simulink model "Channel_estimation_working1"  (R2016b)
settings: Solver=VariableStepAuto  StartTime=0.0  StopTime=10.0  RelTol=1e-3
undefined symbols (not defined in the file or in its folder): physconst
libraries: phasedtxrxlib x7, phasedenvlib x4, dspinverses x2
settings Model: Creator=CHAITRA  LastModifiedBy=ishu

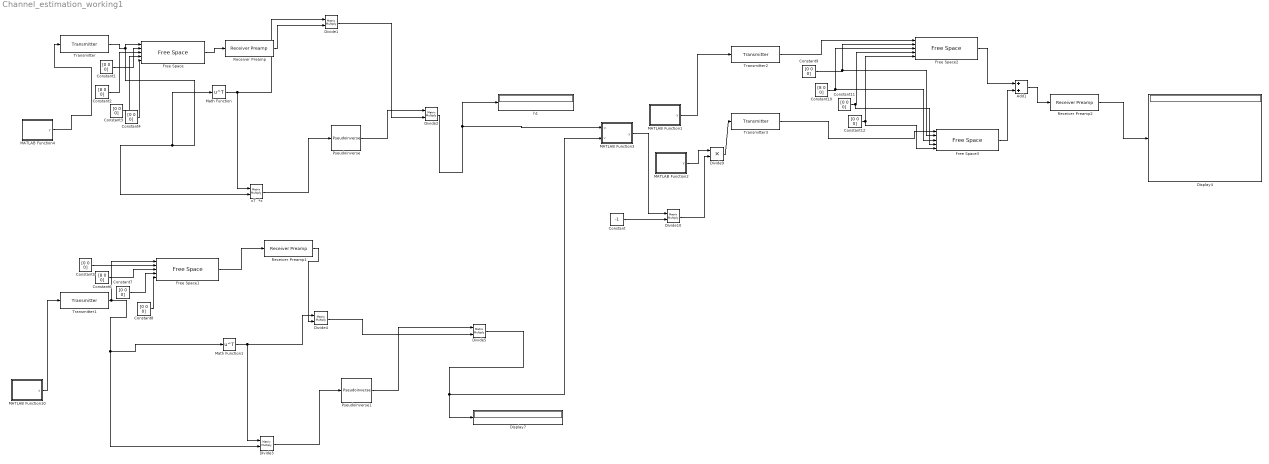
== system Channel_estimation_working1 ==
  Add1 : Sum
  Constant : Constant  Value=-1
  Constant{1,3..5,7..9,11..12} (9 alike) : Constant  Value=[0 0 0]
  Constant10 : Constant  Value=[8 0 0]
  Constant2 : Constant  Value=[8 0 0]
  Constant6 : Constant  Value=[8 0 0]
  Display4 : Display
  Display7 : Display
  Divide{1..5,10} (6 alike) : Product  Multiplication=Matrix(*)
  Divide9 : Product
  Free Space{,1..3} (4 alike) : phasedenvlib/Free Space  PropagationSpeed=physconst( 'LightSpeed' )  OperatingFrequency=3e8  TwoWayPropagation=off  SampleRateFromInputCheckbox=off  SampleRate=100  MaximumDistanceSource=Property  MaximumDistance=10  MaximumNumInputSamplesSource=Auto  MaximumNumInputSamples=1000  SimulateUsing=Interpreted execution
  MATLAB Function1 : MATLAB Function  TreatAsAtomicUnit=on
  MATLAB Function10 : MATLAB Function  TreatAsAtomicUnit=on
  MATLAB Function2 : MATLAB Function  TreatAsAtomicUnit=on
  MATLAB Function3 : MATLAB Function  TreatAsAtomicUnit=on
  MATLAB Function4 : MATLAB Function  TreatAsAtomicUnit=on
  Math Function : Math  Operator=transpose  SaturateOnIntegerOverflow=on
  Math Function1 : Math  Operator=transpose  SaturateOnIntegerOverflow=on
  Pseudoinverse : dspinverses/Pseudoinverse  wanterr=off  SimulateUsing=Interpreted execution
  Pseudoinverse1 : dspinverses/Pseudoinverse  wanterr=off  SimulateUsing=Interpreted execution
  Receiver Preamp : phasedtxrxlib/Receiver Preamp  Gain=20  LossFactor=0  NoiseMethod=Noise power  NoiseFigure=0  ReferenceTemperature=290  SampleRateFromInputCheckbox=on  SampleRate=1e6  NoisePower=0  EnableInputPort=off  PhaseNoiseInputPort=off  SeedSource=Property  Seed=randi(65535,1)  SimulateUsing=Interpreted execution
  Receiver Preamp1 : phasedtxrxlib/Receiver Preamp  Gain=20  LossFactor=0  NoiseMethod=Noise power  NoiseFigure=0  ReferenceTemperature=290  SampleRateFromInputCheckbox=on  SampleRate=1e6  NoisePower=0  EnableInputPort=off  PhaseNoiseInputPort=off  SeedSource=Property  Seed=randi(65535,1)  SimulateUsing=Interpreted execution
  Receiver Preamp2 : phasedtxrxlib/Receiver Preamp  Gain=20  LossFactor=0  NoiseMethod=Noise power  NoiseFigure=0  ReferenceTemperature=290  SampleRateFromInputCheckbox=on  SampleRate=1e6  NoisePower=0  EnableInputPort=off  PhaseNoiseInputPort=off  SeedSource=Property  Seed=randi(65535,1)  SimulateUsing=Interpreted execution
  Transmitter{,1..3} (4 alike) : phasedtxrxlib/Transmitter  PeakPower=5000  Gain=20  LossFactor=0  InUseOutputPort=off  CoherentOnTransmit=on  PhaseNoiseOutputPort=off  SeedSource=Property  Seed=randi(65535,1)  SimulateUsing=Interpreted execution
  "h1 " : Display
  xT  *x : Product  Multiplication=Matrix(*)
  wires:
  Math Function/1 -> xT  *x/1, Divide1/1
  xT  *x/1 -> Pseudoinverse/1
  Divide1/1 -> Divide2/2
  MATLAB Function3/1(y) -> Divide10/1
  MATLAB Function4/1(y) -> Transmitter/1
  Free Space/1 -> Receiver Preamp/1
  Receiver Preamp/1 -> Divide1/2
  Pseudoinverse/1 -> Divide2/1
  Math Function1/1 -> Divide3/1, Divide4/1
  Divide3/1 -> Pseudoinverse1/1
  Divide4/1 -> Divide5/2
  MATLAB Function10/1(y) -> Transmitter1/1
  Receiver Preamp1/1 -> Divide4/2
  Pseudoinverse1/1 -> Divide5/1
  Constant/1 -> Divide10/2
  MATLAB Function1/1(y) -> Transmitter2/1
  Transmitter/1 -> Free Space/1, xT  *x/2, Math Function/1
  Transmitter1/1 -> Free Space1/1, Math Function1/1, Divide3/2
  Divide5/1 -> MATLAB Function3/2(v), Display7/1
  Constant1/1 -> Free Space/2
  Constant2/1 -> Free Space/3
  Constant3/1 -> Free Space/4
  Constant4/1 -> Free Space/5
  Free Space1/1 -> Receiver Preamp1/1
  Constant5/1 -> Free Space1/2
  Constant6/1 -> Free Space1/3
  Constant7/1 -> Free Space1/4
  Constant8/1 -> Free Space1/5
  Divide2/1 -> MATLAB Function3/1(u), "h1 "/1
  Transmitter2/1 -> Free Space2/1
  Constant9/1 -> Free Space3/2, Free Space2/2
  Constant10/1 -> Free Space3/3, Free Space2/3
  Constant11/1 -> Free Space3/4, Free Space2/4
  Constant12/1 -> Free Space3/5, Free Space2/5
  Receiver Preamp2/1 -> Display4/1
  Free Space2/1 -> Add1/1
  Free Space3/1 -> Add1/2
  Add1/1 -> Receiver Preamp2/1
  Transmitter3/1 -> Free Space3/1
  Divide10/1 -> Divide9/2
  MATLAB Function2/1(y) -> Divide9/1
  Divide9/1 -> Transmitter3/1

== matlab function Channel_estimation_working1/MATLAB Function1 ==
  data: y output
function y = fcn()

f = 1;
t = 0:0.01:1;

a = 5*sin(2*pi*f*t);
y = transpose(a);

== matlab function Channel_estimation_working1/MATLAB Function2 ==
  data: y output
function y = fcn()

f = 1;
t = 0:0.01:1;

a = 5*sin(2*pi*f*t);

y = transpose(a);

== matlab function Channel_estimation_working1/MATLAB Function3 ==
  data: u input; y output; v input
function y = fcn(u,v)

%y = ldivide(w,z)
% you can divide each element by the same eleent of other row by
y= u./v ;

== matlab function Channel_estimation_working1/MATLAB Function4 ==
  data: y output
function y = fcn()

f = 1;
t = 0:0.01:1;

a = 5*sin(2*pi*f*t);
y = transpose(a);

== matlab function Channel_estimation_working1/MATLAB Function10 ==
  data: y output
function y = fcn()

f =5
;
t = 0:0.01:1;

a = 5*sin(2*pi*f*t);

y = transpose(a);
